simulink model "PI_VC_vs_UPI_CC_3ph_4w_v2023b"  (R2023b)
settings: Solver=FixedStepDiscrete  StartTime=0.0  StopTime=14  FixedStep=Ts_Power  MaxStep=1e-4  RelTol=1e-3
InitFcn:
  | run PI_VC_vs_UPI_CC_ini;
values from neighbouring files (symbols this model uses):
  C = 4e-6    (= 4e-06)    [PI_OL_vs_PI_CC_ini.m]    (also in PI_VC_vs_UPI_CC_ini.m)
  C_2 = 4e-6    (= 4e-06)    [PI_OL_vs_PI_CC_ini.m]    (also in PI_VC_vs_UPI_CC_ini.m)
  K_i_pll = 1.8/0.00251    (= 717.131474104)    [PI_OL_vs_PI_CC_ini.m]    (also in PI_VC_vs_UPI_CC_ini.m)
  K_p_pll = 1.8    [PI_OL_vs_PI_CC_ini.m]    (also in PI_VC_vs_UPI_CC_ini.m)
  Kp_i = 1*(L_t2 + L_s2)/tau_i    (= 2.5)    [PI_OL_vs_PI_CC_ini.m]    (also in PI_VC_vs_UPI_CC_ini.m)
  Kr_i = 2*(R_t2 + R_s2)/tau_i    (= 157.079632679)    [PI_OL_vs_PI_CC_ini.m]    (also in PI_VC_vs_UPI_CC_ini.m)
  L_line_12_13 = X_line_12_13/(2*pi*50)    (= 0.000798957814321)    [PI_OL_vs_PI_CC_ini.m]    (also in PI_VC_vs_UPI_CC_ini.m)
  L_line_13_14 = X_line_13_14/(2*pi*50)    (= 0.000200535228296)    [PI_OL_vs_PI_CC_ini.m]    (also in PI_VC_vs_UPI_CC_ini.m)
  L_n = L_t2 + L_s2    (= 0.0025)    [PI_OL_vs_PI_CC_ini.m]    (also in PI_VC_vs_UPI_CC_ini.m)
  L_s = 1.25e-3    (= 0.00125)    [PI_OL_vs_PI_CC_ini.m]    (also in PI_VC_vs_UPI_CC_ini.m)
  L_s2 = 1.25e-3    (= 0.00125)    [PI_OL_vs_PI_CC_ini.m]    (also in PI_VC_vs_UPI_CC_ini.m)
  L_t = 1.25e-3    (= 0.00125)    [PI_OL_vs_PI_CC_ini.m]    (also in PI_VC_vs_UPI_CC_ini.m)
  L_t2 = 1.25e-3    (= 0.00125)    [PI_OL_vs_PI_CC_ini.m]    (also in PI_VC_vs_UPI_CC_ini.m)
  omega = 2*pi*f    (= 314.159265359)    [PI_OL_vs_PI_CC_ini.m]    (also in PI_VC_vs_UPI_CC_ini.m)
  params_pi_cc = [S_b,U_b,K_p,T_p,K_q,T_q,X,R]    [PI_OL_vs_PI_CC_ini.m]    (also in PI_VC_vs_UPI_CC_ini.m)
  params_pi_vc = [S_b,U_b,K_p,T_p,K_q,T_q,Xv,Rv]    [PI_OL_vs_PI_CC_ini.m]    (also in PI_VC_vs_UPI_CC_ini.m)
  params_vc_cc = [R_t;L_t;R_s;L_s;K_pi;K_ii;C;K_pv;K_iv]    [PI_OL_vs_PI_CC_ini.m]    (also in PI_VC_vs_UPI_CC_ini.m)
  R_d = 10    [PI_OL_vs_PI_CC_ini.m]    (also in PI_VC_vs_UPI_CC_ini.m)
  R_d2 = 10    [PI_OL_vs_PI_CC_ini.m]    (also in PI_VC_vs_UPI_CC_ini.m)
  R_line_12_13 = (0.06)*Length    (= 0.24)    [PI_OL_vs_PI_CC_ini.m]    (also in PI_VC_vs_UPI_CC_ini.m)
  R_line_13_14 = (0.025)*Length    (= 0.1)    [PI_OL_vs_PI_CC_ini.m]    (also in PI_VC_vs_UPI_CC_ini.m)
  R_n = L_n*omega/10    (= 0.0785398163397)    [PI_OL_vs_PI_CC_ini.m]    (also in PI_VC_vs_UPI_CC_ini.m)
  R_s = L_s*omega/10    (= 0.0392699081699)    [PI_OL_vs_PI_CC_ini.m]    (also in PI_VC_vs_UPI_CC_ini.m)
  R_s2 = L_s*omega/10    (= 0.0392699081699)    [PI_OL_vs_PI_CC_ini.m]    (also in PI_VC_vs_UPI_CC_ini.m)
  R_t = L_t*omega/10    (= 0.0392699081699)    [PI_OL_vs_PI_CC_ini.m]    (also in PI_VC_vs_UPI_CC_ini.m)
  R_t2 = L_t*omega/10    (= 0.0392699081699)    [PI_OL_vs_PI_CC_ini.m]    (also in PI_VC_vs_UPI_CC_ini.m)
  S_b = 20e3    (= 20000)    [PI_OL_vs_PI_CC_ini.m]    (also in PI_VC_vs_UPI_CC_ini.m)
  Ts_Control = 50e-6    (= 5e-05)    [PI_OL_vs_PI_CC_ini.m]    (also in PI_VC_vs_UPI_CC_ini.m)
  Ts_Power = 50e-6    (= 5e-05)    [PI_OL_vs_PI_CC_ini.m]    (also in PI_VC_vs_UPI_CC_ini.m)
  v_dc = 800    [PI_OL_vs_PI_CC_ini.m]    (also in PI_VC_vs_UPI_CC_ini.m)
undefined symbols (not defined in the file or in its folder): DiscIntNeverNeededParam, omega_ref
libraries: spsFirstOrderFilterLib x32, spsUniversalBridgeLib x10, spsThreePhaseSeriesRLCBranchLib x9, spsPowerLib x6, spsThreePhaseVIMeasurementLib x6, eeGeneralControl x5, spsSeriesRLCLoadLib x5, spsRMSLib x4, spsSeriesRLCBranchLib x4, spsPower3phInstantaneousLib x3, spsThreePhaseBreakerLib x3, spsDCVoltageSourceLib x2
(part 3 of 3)

== system PI_VC_vs_UPI_CC_3ph_4w_v2023b/Control UVSG/Control corriente en alpha-beta/Resonant Controller. Impulse invariant/Subsystem1 ==
  error : Inport
  omega_PLL : Inport  Port=2
  Gain1 : Gain  Gain=Kr_i
  MATLAB Function : MATLAB Function  TreatAsAtomicUnit=on
  Unit Delay : UnitDelay  SampleTime=Ts_Control  HasFrameUpgradeWarning=on
  Unit Delay1 : UnitDelay  SampleTime=Ts_Control  HasFrameUpgradeWarning=on
  Unit Delay2 : UnitDelay  SampleTime=Ts_Control  HasFrameUpgradeWarning=on
  y : Outport
  wires:
  Gain1/1 -> MATLAB Function/2(u), Unit Delay2/1
  Unit Delay1/1 -> MATLAB Function/5(y_2)
  Unit Delay/1 -> Unit Delay1/1, MATLAB Function/4(y_1)
  omega_PLL/1 -> MATLAB Function/1(omega_vsg)
  error/1 -> Gain1/1
  MATLAB Function/1(y) -> Unit Delay/1, y/1
  Unit Delay2/1 -> MATLAB Function/3(u_1)

== system PI_VC_vs_UPI_CC_3ph_4w_v2023b/Control UVSG/Reference Computation/Transformadas Park fase/PLL ==
  v_sdq : Inport
  Demux : Demux  Outputs=2
  Discrete-Time Integrator1 : DiscreteIntegrator  SampleTime=Ts_Control  ICPrevOutput=DiscIntNeverNeededParam  ICPrevScaledInput=DiscIntNeverNeededParam
  Integrator with Wrapped State (Discrete or Continuous) : eeGeneralControl/Integrator with Wrapped State (Discrete or Continuous)  LabelModeActiveChoice=Discrete  WrappedStateUpperValue=2*pi  WrappedStateLowerValue=0  x0=0  Ts=Ts_Control
  Ki : Gain  Gain=K_i_pll
  Kp : Gain  Gain=K_p_pll
  Sum : Sum  Inputs=|++
  omega : Outport  VectorParamsAs1DForOutWhenUnconnected=off
  theta : Outport  Port=2  VectorParamsAs1DForOutWhenUnconnected=off
  wires:
  v_sdq/1 -> Demux/1
  Ki/1 -> Discrete-Time Integrator1/1
  Kp/1 -> Sum/1
  Discrete-Time Integrator1/1 -> Sum/2
  Sum/1 -> Integrator with Wrapped State (Discrete or Continuous)/1, omega/1
  Integrator with Wrapped State (Discrete or Continuous)/1 -> [theta], theta/1
  Demux/1 -> Ki/1, Kp/1

== system PI_VC_vs_UPI_CC_3ph_4w_v2023b/Control UVSG/Reference Computation/Transformadas Park fase/alpha-beta_fasea_LPF ==
  u1 : Inport
  omega : Inport  Port=2
  Gain2 : Gain  Gain=2
  MATLAB Function2 : MATLAB Function  TreatAsAtomicUnit=on
  Mux1 : Mux  Inputs=2
  Unit Delay3 : UnitDelay  SampleTime=50e-6  HasFrameUpgradeWarning=on
  Unit Delay4 : UnitDelay  SampleTime=50e-6  HasFrameUpgradeWarning=on
  Unit Delay5 : UnitDelay  SampleTime=50e-6  HasFrameUpgradeWarning=on
  "u1  " : InportShadow
  alpha_beta : Outport
  wires:
  Unit Delay3/1 -> MATLAB Function2/4(y1_k_1)
  MATLAB Function2/1(y1_k) -> Unit Delay3/1
  Unit Delay5/1 -> MATLAB Function2/2(u1_k_1)
  Unit Delay4/1 -> MATLAB Function2/5(y2_k_1)
  MATLAB Function2/2(y2_k) -> Gain2/1, Unit Delay4/1
  "u1  "/1 -> Unit Delay5/1
  omega/1 -> MATLAB Function2/3(omega)
  Gain2/1 -> Mux1/2
  u1/1 -> Mux1/1, MATLAB Function2/1(u1)
  Mux1/1 -> alpha_beta/1

== system PI_VC_vs_UPI_CC_3ph_4w_v2023b/Control UVSG/Reference Computation/Transformadas Park fase/alpha-beta_fasea_LPF1 ==
  u1 : Inport
  omega : Inport  Port=2
  Gain2 : Gain  Gain=2
  MATLAB Function2 : MATLAB Function  TreatAsAtomicUnit=on
  Mux1 : Mux  Inputs=2
  Unit Delay3 : UnitDelay  SampleTime=50e-6  HasFrameUpgradeWarning=on
  Unit Delay4 : UnitDelay  SampleTime=50e-6  HasFrameUpgradeWarning=on
  Unit Delay5 : UnitDelay  SampleTime=50e-6  HasFrameUpgradeWarning=on
  "u1  " : InportShadow
  alpha_beta : Outport
  wires:
  Mux1/1 -> alpha_beta/1
  u1/1 -> MATLAB Function2/1(u1), Mux1/1
  Gain2/1 -> Mux1/2
  omega/1 -> MATLAB Function2/3(omega)
  "u1  "/1 -> Unit Delay5/1
  MATLAB Function2/2(y2_k) -> Unit Delay4/1, Gain2/1
  Unit Delay4/1 -> MATLAB Function2/5(y2_k_1)
  Unit Delay5/1 -> MATLAB Function2/2(u1_k_1)
  MATLAB Function2/1(y1_k) -> Unit Delay3/1
  Unit Delay3/1 -> MATLAB Function2/4(y1_k_1)

== system PI_VC_vs_UPI_CC_3ph_4w_v2023b/Control UVSG/Reference Computation/Transformadas Park fase/alpha-beta_fasea_LPF2 ==
  u1 : Inport
  omega : Inport  Port=2
  Gain2 : Gain  Gain=2
  MATLAB Function2 : MATLAB Function  TreatAsAtomicUnit=on
  Mux1 : Mux  Inputs=2
  Unit Delay3 : UnitDelay  SampleTime=50e-6  HasFrameUpgradeWarning=on
  Unit Delay4 : UnitDelay  SampleTime=50e-6  HasFrameUpgradeWarning=on
  Unit Delay5 : UnitDelay  SampleTime=50e-6  HasFrameUpgradeWarning=on
  "u1  " : InportShadow
  alpha_beta : Outport
  wires:
  Unit Delay3/1 -> MATLAB Function2/4(y1_k_1)
  MATLAB Function2/1(y1_k) -> Unit Delay3/1
  Unit Delay5/1 -> MATLAB Function2/2(u1_k_1)
  Unit Delay4/1 -> MATLAB Function2/5(y2_k_1)
  MATLAB Function2/2(y2_k) -> Gain2/1, Unit Delay4/1
  "u1  "/1 -> Unit Delay5/1
  omega/1 -> MATLAB Function2/3(omega)
  Gain2/1 -> Mux1/2
  u1/1 -> Mux1/1, MATLAB Function2/1(u1)
  Mux1/1 -> alpha_beta/1

== system PI_VC_vs_UPI_CC_3ph_4w_v2023b/Control UVSG/Reference Computation/Transformadas Park fase/alpha-beta_fasea_LPF3 ==
  u1 : Inport
  omega : Inport  Port=2
  Gain2 : Gain  Gain=2
  MATLAB Function2 : MATLAB Function  TreatAsAtomicUnit=on
  Mux1 : Mux  Inputs=2
  Unit Delay3 : UnitDelay  SampleTime=50e-6  HasFrameUpgradeWarning=on
  Unit Delay4 : UnitDelay  SampleTime=50e-6  HasFrameUpgradeWarning=on
  Unit Delay5 : UnitDelay  SampleTime=50e-6  HasFrameUpgradeWarning=on
  "u1  " : InportShadow
  alpha_beta : Outport
  wires:
  Mux1/1 -> alpha_beta/1
  u1/1 -> MATLAB Function2/1(u1), Mux1/1
  Gain2/1 -> Mux1/2
  omega/1 -> MATLAB Function2/3(omega)
  "u1  "/1 -> Unit Delay5/1
  MATLAB Function2/2(y2_k) -> Unit Delay4/1, Gain2/1
  Unit Delay4/1 -> MATLAB Function2/5(y2_k_1)
  Unit Delay5/1 -> MATLAB Function2/2(u1_k_1)
  MATLAB Function2/1(y1_k) -> Unit Delay3/1
  Unit Delay3/1 -> MATLAB Function2/4(y1_k_1)

== system PI_VC_vs_UPI_CC_3ph_4w_v2023b/Control UVSG/Reference Computation/Transformadas Park fase/alpha-beta_fasea_LPF4 ==
  u1 : Inport
  omega : Inport  Port=2
  Gain2 : Gain  Gain=2
  MATLAB Function2 : MATLAB Function  TreatAsAtomicUnit=on
  Mux1 : Mux  Inputs=2
  Unit Delay3 : UnitDelay  SampleTime=50e-6  HasFrameUpgradeWarning=on
  Unit Delay4 : UnitDelay  SampleTime=50e-6  HasFrameUpgradeWarning=on
  Unit Delay5 : UnitDelay  SampleTime=50e-6  HasFrameUpgradeWarning=on
  "u1  " : InportShadow
  alpha_beta : Outport
  wires:
  Unit Delay3/1 -> MATLAB Function2/4(y1_k_1)
  MATLAB Function2/1(y1_k) -> Unit Delay3/1
  Unit Delay5/1 -> MATLAB Function2/2(u1_k_1)
  Unit Delay4/1 -> MATLAB Function2/5(y2_k_1)
  MATLAB Function2/2(y2_k) -> Gain2/1, Unit Delay4/1
  "u1  "/1 -> Unit Delay5/1
  omega/1 -> MATLAB Function2/3(omega)
  Gain2/1 -> Mux1/2
  u1/1 -> Mux1/1, MATLAB Function2/1(u1)
  Mux1/1 -> alpha_beta/1

== system PI_VC_vs_UPI_CC_3ph_4w_v2023b/Control UVSG/Reference Computation/Transformadas Park fase/alpha-beta_fasea_LPF5 ==
  u1 : Inport
  omega : Inport  Port=2
  Gain2 : Gain  Gain=2
  MATLAB Function2 : MATLAB Function  TreatAsAtomicUnit=on
  Mux1 : Mux  Inputs=2
  Unit Delay3 : UnitDelay  SampleTime=50e-6  HasFrameUpgradeWarning=on
  Unit Delay4 : UnitDelay  SampleTime=50e-6  HasFrameUpgradeWarning=on
  Unit Delay5 : UnitDelay  SampleTime=50e-6  HasFrameUpgradeWarning=on
  "u1  " : InportShadow
  alpha_beta : Outport
  wires:
  Mux1/1 -> alpha_beta/1
  u1/1 -> MATLAB Function2/1(u1), Mux1/1
  Gain2/1 -> Mux1/2
  omega/1 -> MATLAB Function2/3(omega)
  "u1  "/1 -> Unit Delay5/1
  MATLAB Function2/2(y2_k) -> Unit Delay4/1, Gain2/1
  Unit Delay4/1 -> MATLAB Function2/5(y2_k_1)
  Unit Delay5/1 -> MATLAB Function2/2(u1_k_1)
  MATLAB Function2/1(y1_k) -> Unit Delay3/1
  Unit Delay3/1 -> MATLAB Function2/4(y1_k_1)

== system PI_VC_vs_UPI_CC_3ph_4w_v2023b/Control UVSG/Reference Computation/VSG_a1/PLL ==
  v_sabc : Inport
  Demux : Demux  Outputs=2
  Discrete-Time Integrator1 : DiscreteIntegrator  InitialCondition=2*pi*50  SampleTime=Ts_Control  ICPrevOutput=DiscIntNeverNeededParam  ICPrevScaledInput=DiscIntNeverNeededParam
  Integrator with Wrapped State (Discrete or Continuous) : eeGeneralControl/Integrator with Wrapped State (Discrete or Continuous)  LabelModeActiveChoice=Discrete  WrappedStateUpperValue=2*pi  WrappedStateLowerValue=0  x0=0  Ts=Ts_Control
  Ki : Gain  Gain=K_i_pll
  Kp : Gain  Gain=K_p_pll
  MATLAB Function1 : MATLAB Function  TreatAsAtomicUnit=on
  Sum : Sum  Inputs=|++
  omega : Outport  VectorParamsAs1DForOutWhenUnconnected=off
  theta : Outport  Port=2  VectorParamsAs1DForOutWhenUnconnected=off
  wires:
  MATLAB Function1/1(dq) -> Demux/1
  v_sabc/1 -> MATLAB Function1/2(abc)
  [theta] -> MATLAB Function1/1(theta)
  Ki/1 -> Discrete-Time Integrator1/1
  Kp/1 -> Sum/1
  Discrete-Time Integrator1/1 -> Sum/2
  Sum/1 -> Integrator with Wrapped State (Discrete or Continuous)/1, omega/1
  Integrator with Wrapped State (Discrete or Continuous)/1 -> [theta], theta/1
  Demux/1 -> Ki/1, Kp/1

== system PI_VC_vs_UPI_CC_3ph_4w_v2023b/Control UVSG/Reference Computation/VSG_a2/PLL ==
  v_sabc : Inport
  Demux : Demux  Outputs=2
  Discrete-Time Integrator1 : DiscreteIntegrator  InitialCondition=2*pi*50  SampleTime=Ts_Control  ICPrevOutput=DiscIntNeverNeededParam  ICPrevScaledInput=DiscIntNeverNeededParam
  Integrator with Wrapped State (Discrete or Continuous) : eeGeneralControl/Integrator with Wrapped State (Discrete or Continuous)  LabelModeActiveChoice=Discrete  WrappedStateUpperValue=2*pi  WrappedStateLowerValue=0  x0=0  Ts=Ts_Control
  Ki : Gain  Gain=K_i_pll
  Kp : Gain  Gain=K_p_pll
  MATLAB Function1 : MATLAB Function  TreatAsAtomicUnit=on
  Sum : Sum  Inputs=|++
  omega : Outport  VectorParamsAs1DForOutWhenUnconnected=off
  theta : Outport  Port=2  VectorParamsAs1DForOutWhenUnconnected=off
  wires:
  MATLAB Function1/1(dq) -> Demux/1
  v_sabc/1 -> MATLAB Function1/2(abc)
  [theta] -> MATLAB Function1/1(theta)
  Ki/1 -> Discrete-Time Integrator1/1
  Kp/1 -> Sum/1
  Discrete-Time Integrator1/1 -> Sum/2
  Sum/1 -> Integrator with Wrapped State (Discrete or Continuous)/1, omega/1
  Integrator with Wrapped State (Discrete or Continuous)/1 -> [theta], theta/1
  Demux/1 -> Ki/1, Kp/1

== matlab function PI_VC_vs_UPI_CC_3ph_4w_v2023b/Control PI_VC/Voltage Control ==
  data: v_cdq_ref input; i_sdq input; i_tdq_ref output size=2; v_cdq input; omega input; params input; x input; dx output
function [i_tdq_ref,dx] = ctrl_vsc(v_cdq_ref,i_sdq,v_cdq,omega,params,x)

% parameters
C = params(7);
K_pv = params(8);
K_iv = params(9);

%References
v_cd_ref = v_cdq_ref(1);
v_cq_ref = v_cdq_ref(2);

i_sd = i_sdq(1);
i_sq = i_sdq(2);
v_cd = v_cdq(1);
v_cq = v_cdq(2);

% from the integrator to the states
xi_vcd = x(1);
xi_vcq = x(2);


% auxiliar
e_vcd = v_cd_ref - v_cd;
e_vcq = v_cq_ref - v_cq;

% derivatives
dxi_vcd = e_vcd;
dxi_vcq = e_vcq;


% auxiliar
u_d = K_pv*e_vcd + K_iv*xi_vcd;
u_q = K_pv*e_vcq + K_iv*xi_vcq;

% outputs
i_td_ref = (u_d - C*omega*v_cq + i_sd);
i_tq_ref = (u_q + C*omega*v_cd + i_sq);
i_tdq_ref = [i_td_ref ; i_tq_ref];


% from derivatives to the integrator
dx = [dxi_vcd;dxi_vcq];

== matlab function PI_VC_vs_UPI_CC_3ph_4w_v2023b/Control UVSG/Control corriente en alpha-beta/Resonant Controller. Impulse Invariant ==
  data: v_dc input size=1; v_salbe input size=2; eta_albe output size=2; eta_n output; u output size=2; i_sal_ref input size=1; y output size=2; u_n output; i_sbe_ref input size=1; i_salbe input size=2; omega input size=1; i_n input; i_n_ref input; u_aux_1 input size=2; y_aux_1 input size=2; y_aux_2 input size=2; u_aux_1_n input; y_aux_1_n input; y_aux_2_n input; Ts_Control parameter; Kp_i parameter; Kr_i parameter; y_aux_n output
function [eta_albe,eta_n,u,y,u_n,y_aux_n] = fcn(v_dc,v_salbe,i_sal_ref,i_sbe_ref,i_salbe,omega,i_n,i_n_ref,u_aux_1,y_aux_1,y_aux_2, u_aux_1_n, y_aux_1_n,y_aux_2_n,Ts_Control,Kp_i, Kr_i)

%Parameters

%Measurements
i_sal = i_salbe(1);
i_sbe = i_salbe(2);
v_sal = v_salbe(1);
v_sbe = v_salbe(2);

%error
e_sal = i_sal_ref - i_sal;
e_sbe = i_sbe_ref - i_sbe;

e_n = i_n_ref - i_n;


%Auxiliar
u_al = Kr_i*e_sal;
u_be = Kr_i*e_sbe;
u = [u_al;u_be];

u_n = Kr_i*e_n;

u_aux_1_al = u_aux_1(1);
u_aux_1_be = u_aux_1(2);

y_aux_1_al = y_aux_1(1);
y_aux_1_be = y_aux_1(2);

y_aux_2_al = y_aux_2(1);
y_aux_2_be = y_aux_2(2);


%Resonant controller impulse invariant
Ts = Ts_Control;
y_aux_al = u_al*Ts - u_aux_1_al*Ts*cos(omega*Ts) + 2*y_aux_1_al*cos(omega*Ts) - y_aux_2_al;
y_aux_be = u_be*Ts - u_aux_1_be*Ts*cos(omega*Ts) + 2*y_aux_1_be*cos(omega*Ts) - y_aux_2_be;

y_aux_n = u_n*Ts - u_aux_1_n*Ts*cos(omega*Ts) + 2*y_aux_1_n*cos(omega*Ts) - y_aux_2_n;

y = [y_aux_al;y_aux_be];


y_al = Kp_i*e_sal + y_aux_al;
y_be = Kp_i*e_sbe + y_aux_be;

y_n = Kp_i*e_n + y_aux_n;

%Outputs
eta_al = (y_al + v_sal)*2/v_dc;
eta_be = (y_be + v_sbe)*2/v_dc;

eta_n = (y_n)*2/v_dc;

eta_albe = [eta_al;eta_be];

== matlab function PI_VC_vs_UPI_CC_3ph_4w_v2023b/Control UVSG/Control corriente en alpha-beta/Resonant Controller. Impulse invariant/Subsystem/MATLAB Function ==
  data: omega_vsg input; y output; Ts_Control parameter; u input; u_1 input; y_1 input; y_2 input
function y  = fcn(omega_vsg, Ts_Control,u,u_1,y_1,y_2)

Ts = Ts_Control;
y = u*Ts - u_1*Ts*cos(omega_vsg*Ts) + 2*y_1*cos(omega_vsg*Ts) - y_2;

== matlab function PI_VC_vs_UPI_CC_3ph_4w_v2023b/Control UVSG/Control corriente en alpha-beta/Resonant Controller. Impulse invariant/Subsystem1/MATLAB Function ==
  data: omega_vsg input; y output; Ts_Control parameter; u input; u_1 input; y_1 input; y_2 input
function y  = fcn(omega_vsg, Ts_Control,u,u_1,y_1,y_2)

Ts = Ts_Control;
y = u*Ts - u_1*Ts*cos(omega_vsg*Ts) + 2*y_1*cos(omega_vsg*Ts) - y_2;

== matlab function PI_VC_vs_UPI_CC_3ph_4w_v2023b/Control UVSG/PARK_PLL/MATLAB Function1 ==
  data: theta input size=1; dq output; abc input
function dq  = fcn(theta,abc)
%#codegen

T_p = 2.0/3.0*[[ cos(theta), cos(theta-2.0/3.0*pi), cos(theta+2.0/3.0*pi)];
               [-sin(theta),-sin(theta-2.0/3.0*pi),-sin(theta+2.0/3.0*pi)]];
           
dq=T_p*abc;

== matlab function PI_VC_vs_UPI_CC_3ph_4w_v2023b/Control UVSG/PARK_PLL/MATLAB Function2 ==
  data: theta input size=1; dq output; abc input
function dq  = fcn(theta,abc)
%#codegen

T_p = 2.0/3.0*[[ cos(theta), cos(theta-2.0/3.0*pi), cos(theta+2.0/3.0*pi)];
               [-sin(theta),-sin(theta-2.0/3.0*pi),-sin(theta+2.0/3.0*pi)]];
           
dq=T_p*abc;

== matlab function PI_VC_vs_UPI_CC_3ph_4w_v2023b/Control UVSG/Control corriente en alpha-beta/Resonant Controller. Impulse Invariant1 ==
  data: v_dc input size=1; v_salbe input size=2; eta_albe output size=2; eta_n output; u output size=2; i_sal_ref input size=1; y output size=2; u_n output; i_sbe_ref input size=1; i_salbe input size=2; omega input size=1; i_n input; i_n_ref input; u_aux_1 input size=2; y_aux_1 input size=2; y_aux_2 input size=2; u_aux_1_n input; y_aux_1_n input; y_aux_2_n input; Ts_Control parameter; Kp_i parameter; Kr_i parameter; y_aux_n output
function [eta_albe,eta_n,u,y,u_n,y_aux_n] = fcn(v_dc,v_salbe,i_sal_ref,i_sbe_ref,i_salbe,omega,i_n,i_n_ref,u_aux_1,y_aux_1,y_aux_2, u_aux_1_n, y_aux_1_n,y_aux_2_n,Ts_Control,Kp_i, Kr_i)

%Parameters

%Measurements
i_sal = i_salbe(1);
i_sbe = i_salbe(2);
v_sal = v_salbe(1);
v_sbe = v_salbe(2);

%error
e_sal = i_sal_ref - i_sal;
e_sbe = i_sbe_ref - i_sbe;

e_n = i_n_ref - i_n;


%Auxiliar
u_al = Kr_i*e_sal;
u_be = Kr_i*e_sbe;
u = [u_al;u_be];

u_n = Kr_i*e_n;

u_aux_1_al = u_aux_1(1);
u_aux_1_be = u_aux_1(2);

y_aux_1_al = y_aux_1(1);
y_aux_1_be = y_aux_1(2);

y_aux_2_al = y_aux_2(1);
y_aux_2_be = y_aux_2(2);


%Resonant controller impulse invariant
Ts = Ts_Control;
y_aux_al = u_al*Ts - u_aux_1_al*Ts*cos(omega*Ts) + 2*y_aux_1_al*cos(omega*Ts) - y_aux_2_al;
y_aux_be = u_be*Ts - u_aux_1_be*Ts*cos(omega*Ts) + 2*y_aux_1_be*cos(omega*Ts) - y_aux_2_be;

y_aux_n = u_n*Ts - u_aux_1_n*Ts*cos(omega*Ts) + 2*y_aux_1_n*cos(omega*Ts) - y_aux_2_n;

y = [y_aux_al;y_aux_be];


y_al = Kp_i*e_sal + y_aux_al;
y_be = Kp_i*e_sbe + y_aux_be;

y_n = Kp_i*e_n + y_aux_n;

%Outputs
eta_al = (y_al + v_sal)*2/v_dc;
eta_be = (y_be + v_sbe)*2/v_dc;

eta_n = (y_n)*2/v_dc;

eta_albe = [eta_al;eta_be];

== matlab function PI_VC_vs_UPI_CC_3ph_4w_v2023b/Control UVSG/PARK_PLL/MATLAB Function3 ==
  data: theta input size=1; dq output; abc input
function dq  = fcn(theta,abc)
%#codegen

T_p = 2.0/3.0*[[ cos(theta), cos(theta-2.0/3.0*pi), cos(theta+2.0/3.0*pi)];
               [-sin(theta),-sin(theta-2.0/3.0*pi),-sin(theta+2.0/3.0*pi)]];
           
dq=T_p*abc;

== matlab function PI_VC_vs_UPI_CC_3ph_4w_v2023b/Control UVSG/PARK_PLL/MATLAB Function5 ==
  data: theta input size=1; abc output size=3; dq input
function abc  = fcn(theta,dq)
%#codegen

T_p_inv = [[            cos(theta),            -sin(theta)];
           [ cos(theta-2.0/3.0*pi), -sin(theta-2.0/3.0*pi)];
           [ cos(theta+2.0/3.0*pi), -sin(theta+2.0/3.0*pi)]];
           
abc=T_p_inv*dq;

== matlab function PI_VC_vs_UPI_CC_3ph_4w_v2023b/Control UVSG/PARK_PLL/PLL/MATLAB Function1 ==
  data: theta input size=1; dq output; abc input
function dq  = fcn(theta,abc)
%#codegen

T_p = 2.0/3.0*[[ cos(theta), cos(theta-2.0/3.0*pi), cos(theta+2.0/3.0*pi)];
               [-sin(theta),-sin(theta-2.0/3.0*pi),-sin(theta+2.0/3.0*pi)]];
           
dq=T_p*abc;

== matlab function PI_VC_vs_UPI_CC_3ph_4w_v2023b/Control UVSG/Reference Computation/MATLAB Function1 ==
  data: albe input size=2; a output size=1
function a  = fcn(albe)
%#codegen
theta = 0;
a=cos(theta)*albe(1) - sin(theta)*albe(2) ;

== matlab function PI_VC_vs_UPI_CC_3ph_4w_v2023b/Control UVSG/Reference Computation/MATLAB Function2 ==
  data: albe input size=2; a output size=1
function a  = fcn(albe)
%#codegen
theta = 0;
a=cos(theta)*albe(1) - sin(theta)*albe(2) ;

== matlab function PI_VC_vs_UPI_CC_3ph_4w_v2023b/Control UVSG/Reference Computation/MATLAB Function5 ==
  data: albe input size=2; a output size=1
function a  = fcn(albe)
%#codegen
theta = 0;
a=cos(theta)*albe(1) - sin(theta)*albe(2) ;

== matlab function PI_VC_vs_UPI_CC_3ph_4w_v2023b/Control UVSG/Reference Computation/Transformadas Park fase/MATLAB Function1 ==
  data: alpha_beta input size=2; dq output; theta input
function dq = fcn(alpha_beta,theta)
alpha = alpha_beta(1);
beta = alpha_beta(2);

d= alpha*cos(theta)+ beta*sin(theta);
q= -alpha*sin(theta) + beta*cos(theta);
dq = [d;q];

== matlab function PI_VC_vs_UPI_CC_3ph_4w_v2023b/Control UVSG/Reference Computation/Transformadas Park fase/MATLAB Function2 ==
  data: alpha_beta input size=2; dq output; theta input
function dq = fcn(alpha_beta,theta)
alpha = alpha_beta(1);
beta = alpha_beta(2);

d= alpha*cos(theta)+ beta*sin(theta);
q= -alpha*sin(theta) + beta*cos(theta);
dq = [d;q];

== matlab function PI_VC_vs_UPI_CC_3ph_4w_v2023b/Control UVSG/Reference Computation/Transformadas Park fase/MATLAB Function3 ==
  data: alpha_beta input size=2; dq output; theta input
function dq = fcn(alpha_beta,theta)
alpha = alpha_beta(1);
beta = alpha_beta(2);

d= alpha*cos(theta)+ beta*sin(theta);
q= -alpha*sin(theta) + beta*cos(theta);
dq = [d;q];

== matlab function PI_VC_vs_UPI_CC_3ph_4w_v2023b/Control PI_VC/Current Control ==
  data: i_tdq_ref input; i_tdq input; eta_dq output size=2; v_cdq input; v_dc input; omega input; params input; x input; dx output
function [eta_dq,dx] = ctrl_vsc(i_tdq_ref,i_tdq,v_cdq,v_dc,omega,params,x)

% parameters
L_t = params(2);
K_pi = params(5);
K_ii = params(6);

%References
i_td_ref = i_tdq_ref(1);
i_tq_ref = i_tdq_ref(2);

i_td = i_tdq(1);
i_tq = i_tdq(2);
v_cd = v_cdq(1);
v_cq = v_cdq(2);

% from the integrator to the states
xi_itd = x(1);
xi_itq = x(2);


% auxiliar
e_itd = i_td_ref - i_td;
e_itq = i_tq_ref - i_tq;

% derivatives
dxi_itd = e_itd;
dxi_itq = e_itq;


% auxiliar
u_d = K_pi*e_itd + K_ii*xi_itd;
u_q = K_pi*e_itq + K_ii*xi_itq;
L = L_t;

% outputs
eta_d = 2/v_dc*(u_d - L*omega*i_tq + v_cd);
eta_q = 2/v_dc*(u_q + L*omega*i_td + v_cq);
eta_dq = [eta_d ; eta_q];


% from derivatives to the integrator
dx = [dxi_itd;dxi_itq];

== matlab function PI_VC_vs_UPI_CC_3ph_4w_v2023b/Control UVSG/Reference Computation/Transformadas Park fase/alpha-beta_fasea_LPF/MATLAB Function2 ==
  data: u1 input; u1_k_1 input; omega input; y1_k_1 input; y1_k output; y2_k_1 input; y2_k output
function [y1_k,y2_k]  = fcn(u1,u1_k_1,omega,y1_k_1,y2_k_1)


Ts_Control = 50e-6;
%y = x
%y1_k = (u1*omega + exp(-omega)*y1_k_1);
y1_k = ((u1 + u1_k_1)*omega*Ts_Control - (omega*Ts_Control-2)*y1_k_1)/(omega*Ts_Control + 2);

u2 = y1_k;
u2_k_1 = y1_k_1;

%y2_k = (u2*omega + exp(-omega)*y2_k_1);
y2_k = ((u2 + u2_k_1)*omega*Ts_Control - (omega*Ts_Control-2)*y2_k_1)/(omega*Ts_Control + 2);

== matlab function PI_VC_vs_UPI_CC_3ph_4w_v2023b/Control UVSG/Reference Computation/Transformadas Park fase/alpha-beta_fasea_LPF1/MATLAB Function2 ==
  data: u1 input; u1_k_1 input; omega input; y1_k_1 input; y1_k output; y2_k_1 input; y2_k output
function [y1_k,y2_k]  = fcn(u1,u1_k_1,omega,y1_k_1,y2_k_1)


Ts_Control = 50e-6;
%y = x
%y1_k = (u1*omega + exp(-omega)*y1_k_1);
y1_k = ((u1 + u1_k_1)*omega*Ts_Control - (omega*Ts_Control-2)*y1_k_1)/(omega*Ts_Control + 2);

u2 = y1_k;
u2_k_1 = y1_k_1;

%y2_k = (u2*omega + exp(-omega)*y2_k_1);
y2_k = ((u2 + u2_k_1)*omega*Ts_Control - (omega*Ts_Control-2)*y2_k_1)/(omega*Ts_Control + 2);

== matlab function PI_VC_vs_UPI_CC_3ph_4w_v2023b/Control UVSG/Reference Computation/Transformadas Park fase/alpha-beta_fasea_LPF2/MATLAB Function2 ==
  data: u1 input; u1_k_1 input; omega input; y1_k_1 input; y1_k output; y2_k_1 input; y2_k output
function [y1_k,y2_k]  = fcn(u1,u1_k_1,omega,y1_k_1,y2_k_1)


Ts_Control = 50e-6;
%y = x
%y1_k = (u1*omega + exp(-omega)*y1_k_1);
y1_k = ((u1 + u1_k_1)*omega*Ts_Control - (omega*Ts_Control-2)*y1_k_1)/(omega*Ts_Control + 2);

u2 = y1_k;
u2_k_1 = y1_k_1;

%y2_k = (u2*omega + exp(-omega)*y2_k_1);
y2_k = ((u2 + u2_k_1)*omega*Ts_Control - (omega*Ts_Control-2)*y2_k_1)/(omega*Ts_Control + 2);

== matlab function PI_VC_vs_UPI_CC_3ph_4w_v2023b/Control UVSG/Reference Computation/Transformadas Park fase/MATLAB Function ==
  data: v_salbe_a input size=2; p output; i_salbe_a input size=2; q output
function [p,q] = fcn(v_salbe_a,i_salbe_a)

vs_al = v_salbe_a(1);
vs_be = v_salbe_a(2);
is_al = i_salbe_a(1);
is_be = i_salbe_a(2);
p=3/2*(vs_al*is_al + vs_be*is_be);
q=-3/2*(vs_al*is_be - vs_be*is_al);

== matlab function PI_VC_vs_UPI_CC_3ph_4w_v2023b/Control UVSG/Reference Computation/Transformadas Park fase/MATLAB Function4 ==
  data: v_salbe_a input size=2; p output; i_salbe_a input size=2; q output
function [p,q] = fcn(v_salbe_a,i_salbe_a)

vs_al = v_salbe_a(1);
vs_be = v_salbe_a(2);
is_al = i_salbe_a(1);
is_be = i_salbe_a(2);
p=3/2*(vs_al*is_al + vs_be*is_be);
q=-3/2*(vs_al*is_be - vs_be*is_al);

== matlab function PI_VC_vs_UPI_CC_3ph_4w_v2023b/Control UVSG/Reference Computation/Transformadas Park fase/MATLAB Function5 ==
  data: v_salbe_a input size=2; p output; i_salbe_a input size=2; q output
function [p,q] = fcn(v_salbe_a,i_salbe_a)

vs_al = v_salbe_a(1);
vs_be = v_salbe_a(2);
is_al = i_salbe_a(1);
is_be = i_salbe_a(2);
p=3/2*(vs_al*is_al + vs_be*is_be);
q=-3/2*(vs_al*is_be - vs_be*is_al);

== matlab function PI_VC_vs_UPI_CC_3ph_4w_v2023b/Control UVSG/Reference Computation/Transformadas Park fase/alpha-beta_fasea_LPF3/MATLAB Function2 ==
  data: u1 input; u1_k_1 input; omega input; y1_k_1 input; y1_k output; y2_k_1 input; y2_k output
function [y1_k,y2_k]  = fcn(u1,u1_k_1,omega,y1_k_1,y2_k_1)


Ts_Control = 50e-6;
%y = x
%y1_k = (u1*omega + exp(-omega)*y1_k_1);
y1_k = ((u1 + u1_k_1)*omega*Ts_Control - (omega*Ts_Control-2)*y1_k_1)/(omega*Ts_Control + 2);

u2 = y1_k;
u2_k_1 = y1_k_1;

%y2_k = (u2*omega + exp(-omega)*y2_k_1);
y2_k = ((u2 + u2_k_1)*omega*Ts_Control - (omega*Ts_Control-2)*y2_k_1)/(omega*Ts_Control + 2);

== matlab function PI_VC_vs_UPI_CC_3ph_4w_v2023b/Control UVSG/Reference Computation/Transformadas Park fase/alpha-beta_fasea_LPF4/MATLAB Function2 ==
  data: u1 input; u1_k_1 input; omega input; y1_k_1 input; y1_k output; y2_k_1 input; y2_k output
function [y1_k,y2_k]  = fcn(u1,u1_k_1,omega,y1_k_1,y2_k_1)


Ts_Control = 50e-6;
%y = x
%y1_k = (u1*omega + exp(-omega)*y1_k_1);
y1_k = ((u1 + u1_k_1)*omega*Ts_Control - (omega*Ts_Control-2)*y1_k_1)/(omega*Ts_Control + 2);

u2 = y1_k;
u2_k_1 = y1_k_1;

%y2_k = (u2*omega + exp(-omega)*y2_k_1);
y2_k = ((u2 + u2_k_1)*omega*Ts_Control - (omega*Ts_Control-2)*y2_k_1)/(omega*Ts_Control + 2);

== matlab function PI_VC_vs_UPI_CC_3ph_4w_v2023b/Control UVSG/Reference Computation/Transformadas Park fase/alpha-beta_fasea_LPF5/MATLAB Function2 ==
  data: u1 input; u1_k_1 input; omega input; y1_k_1 input; y1_k output; y2_k_1 input; y2_k output
function [y1_k,y2_k]  = fcn(u1,u1_k_1,omega,y1_k_1,y2_k_1)


Ts_Control = 50e-6;
%y = x
%y1_k = (u1*omega + exp(-omega)*y1_k_1);
y1_k = ((u1 + u1_k_1)*omega*Ts_Control - (omega*Ts_Control-2)*y1_k_1)/(omega*Ts_Control + 2);

u2 = y1_k;
u2_k_1 = y1_k_1;

%y2_k = (u2*omega + exp(-omega)*y2_k_1);
y2_k = ((u2 + u2_k_1)*omega*Ts_Control - (omega*Ts_Control-2)*y2_k_1)/(omega*Ts_Control + 2);

== matlab function PI_VC_vs_UPI_CC_3ph_4w_v2023b/Control UVSG/Reference Computation/VSG_a/MATLAB Function1 ==
  data: theta input size=1; dq output; abc input
function dq  = fcn(theta,abc)
%#codegen

T_p = 2.0/3.0*[[ cos(theta), cos(theta-2.0/3.0*pi), cos(theta+2.0/3.0*pi)];
               [-sin(theta),-sin(theta-2.0/3.0*pi),-sin(theta+2.0/3.0*pi)]];
           
dq=T_p*abc;

== matlab function PI_VC_vs_UPI_CC_3ph_4w_v2023b/Control UVSG/Reference Computation/VSG_a/MATLAB Function2 ==
  data: alpha_beta input size=2; dq output; theta input
function dq = fcn(alpha_beta,theta)
alpha = alpha_beta(1);
beta = alpha_beta(2);

d= alpha*cos(theta)+ beta*sin(theta);
q= -alpha*sin(theta) + beta*cos(theta);
dq = [d;q];

== matlab function PI_VC_vs_UPI_CC_3ph_4w_v2023b/Control UVSG/Reference Computation/VSG_a/MATLAB Function3 ==
  data: theta input size=1; abc output size=3; dq input
function abc  = fcn(theta,dq)
%#codegen

T_p_inv = [[            cos(theta),            -sin(theta)];
           [ cos(theta-2.0/3.0*pi), -sin(theta-2.0/3.0*pi)];
           [ cos(theta+2.0/3.0*pi), -sin(theta+2.0/3.0*pi)]];
           
abc=T_p_inv*dq;

== matlab function PI_VC_vs_UPI_CC_3ph_4w_v2023b/Control UVSG/Reference Computation/VSG_a/MATLAB Function4 ==
  data: alpha_beta input size=2; dq output; theta input
function dq = fcn(alpha_beta,theta)
alpha = alpha_beta(1);
beta = alpha_beta(2);

d= alpha*cos(theta)+ beta*sin(theta);
q= -alpha*sin(theta) + beta*cos(theta);
dq = [d;q];

== matlab function PI_VC_vs_UPI_CC_3ph_4w_v2023b/Control UVSG/Reference Computation/VSG_a/VSG ==
  data: p_m_ref input; q_s_ref input; p input; q input; i_sdq input; i_sdq_ref output size=2; omega_rads output; v_sdq input; params input; omega_base input; x input; dx output
function [i_sdq_ref,omega_rads,dx] = ctrl_3(p_m_ref,q_s_ref,p,q,i_sdq,v_sdq,params,omega_base,x)
%Initialization
i_sdq_ref = [0;0];
fault_flag = 0;
e_0 = 1.0;

% parameters
S_b = params(1);
U_b = params(2);
K_p = params(3);
T_p = params(4);
K_q = params(5);
T_q = params(6);
X = params(7);
R = params(8);

%Base value
I_b = S_b/(sqrt(3)*U_b);
I_bdq = I_b*sqrt(2); 
U_bdq = U_b*(sqrt(2/3));

%Current and voltage in pu
v_sd = v_sdq(1)/U_bdq; % input in SI that is coverted to pu
v_sq = v_sdq(2)/U_bdq; % input in SI that is coverted to pu
i_sd = i_sdq(1)/I_bdq; % input in SI that is coverted to pu
i_sq = i_sdq(2)/I_bdq; % input in SI that is coverted to pu
%Active power en pu
p_s = i_sd*v_sd + i_sq*v_sq; % pu
q_s = i_sd*v_sq - i_sq*v_sd; % pu 

% from the integrator to the states
phi  = x(1);
xi_p = x(2);
xi_q = x(3);
omega_fil = x(4);

%error of active and reactive power
epsilon_p = (p_m_ref - p_s)*(1.0-fault_flag);
epsilon_q = q_s_ref - q_s;

%omega VSG
omega = K_p*(epsilon_p + xi_p/T_p) + omega_base; 
omega_rads = 2.0*pi*50.0*omega;
%Derivative outputs
dphi =  omega_rads;
dxi_p = epsilon_p;
dxi_q = epsilon_q; 
domega_rads = 1.0/1.0*(2.0*pi*50.0*omega - omega_fil);

%Voltage increase
DV =   K_q*(epsilon_q + xi_q/T_q); 

%Saturation of DV
DV_sat = DV;
if DV_sat > 0.1 
    DV_sat = 0.1;
    dxi_q = 0.0;
end
if DV_sat < -0.1 
    DV_sat = -0.1;
    dxi_q = 0.0;
end   

%Electromotive force of VSG
e = e_0 + DV_sat; 

%Virtual impdance
i_sd = -(X*e + R*v_sd + X*v_sq)/(R^2 + X^2);
i_sq = -(R*e + R*v_sq - X*v_sd)/(R^2 + X^2);

%Current references in A
i_sdq_ref(1) = i_sd*I_bdq;
i_sdq_ref(2) = i_sq*I_bdq;


% from derivatives to the integrator
dx = [dphi;dxi_p;dxi_q;domega_rads];

== matlab function PI_VC_vs_UPI_CC_3ph_4w_v2023b/Control PI_VC/PLL/MATLAB Function1 ==
  data: theta input size=1; dq output; abc input
function dq  = fcn(theta,abc)
%#codegen

T_p = 2.0/3.0*[[ cos(theta), cos(theta-2.0/3.0*pi), cos(theta+2.0/3.0*pi)];
               [-sin(theta),-sin(theta-2.0/3.0*pi),-sin(theta+2.0/3.0*pi)]];
           
dq=T_p*abc;

== matlab function PI_VC_vs_UPI_CC_3ph_4w_v2023b/Control UVSG/Reference Computation/Transformadas Park fase/MATLAB Function6 ==
  data: i_sabc input; pa output; v_sabc input; qa output; pb output; qb output; pc output; qc output
function [pa,qa,pb,qb,pc,qc] = fcn(i_sabc,v_sabc)

ia = i_sabc(1);
ib = i_sabc(2);
ic = i_sabc(3);

va = v_sabc(1);
vb = v_sabc(2);
vc = v_sabc(3);

pa = ia*va;
qa = 1/sqrt(3)*ia*(vb - vc);

pb = ib*vb;
qb = 1/sqrt(3)*ib*(vc -va);

pc = ic*vc;
qc = 1/sqrt(3)*ic*(va -vb);

== matlab function PI_VC_vs_UPI_CC_3ph_4w_v2023b/Control UVSG/Reference Computation/VSG_a1/MATLAB Function1 ==
  data: theta input size=1; dq output; abc input
function dq  = fcn(theta,abc)
%#codegen

T_p = 2.0/3.0*[[ cos(theta), cos(theta-2.0/3.0*pi), cos(theta+2.0/3.0*pi)];
               [-sin(theta),-sin(theta-2.0/3.0*pi),-sin(theta+2.0/3.0*pi)]];
           
dq=T_p*abc;

== matlab function PI_VC_vs_UPI_CC_3ph_4w_v2023b/Control UVSG/Reference Computation/VSG_a1/MATLAB Function2 ==
  data: alpha_beta input size=2; dq output; theta input
function dq = fcn(alpha_beta,theta)
alpha = alpha_beta(1);
beta = alpha_beta(2);

d= alpha*cos(theta)+ beta*sin(theta);
q= -alpha*sin(theta) + beta*cos(theta);
dq = [d;q];

== matlab function PI_VC_vs_UPI_CC_3ph_4w_v2023b/Control UVSG/Reference Computation/VSG_a1/MATLAB Function3 ==
  data: theta input size=1; abc output size=3; dq input
function abc  = fcn(theta,dq)
%#codegen

T_p_inv = [[            cos(theta),            -sin(theta)];
           [ cos(theta-2.0/3.0*pi), -sin(theta-2.0/3.0*pi)];
           [ cos(theta+2.0/3.0*pi), -sin(theta+2.0/3.0*pi)]];
           
abc=T_p_inv*dq;

== matlab function PI_VC_vs_UPI_CC_3ph_4w_v2023b/Control UVSG/Reference Computation/VSG_a1/MATLAB Function4 ==
  data: alpha_beta input size=2; dq output; theta input
function dq = fcn(alpha_beta,theta)
alpha = alpha_beta(1);
beta = alpha_beta(2);

d= alpha*cos(theta)+ beta*sin(theta);
q= -alpha*sin(theta) + beta*cos(theta);
dq = [d;q];

== matlab function PI_VC_vs_UPI_CC_3ph_4w_v2023b/Control UVSG/Reference Computation/VSG_a1/VSG ==
  data: p_m_ref input; q_s_ref input; p input; q input; i_sdq input; i_sdq_ref output size=2; omega_rads output; v_sdq input; params input; omega_base input; x input; dx output
function [i_sdq_ref,omega_rads,dx] = ctrl_3(p_m_ref,q_s_ref,p,q,i_sdq,v_sdq,params,omega_base,x)
%Initialization
i_sdq_ref = [0;0];
fault_flag = 0;
e_0 = 1.0;

% parameters
S_b = params(1);
U_b = params(2);
K_p = params(3);
T_p = params(4);
K_q = params(5);
T_q = params(6);
X = params(7);
R = params(8);

%Base value
I_b = S_b/(sqrt(3)*U_b);
I_bdq = I_b*sqrt(2); 
U_bdq = U_b*(sqrt(2/3));

%Current and voltage in pu
v_sd = v_sdq(1)/U_bdq; % input in SI that is coverted to pu
v_sq = v_sdq(2)/U_bdq; % input in SI that is coverted to pu
i_sd = i_sdq(1)/I_bdq; % input in SI that is coverted to pu
i_sq = i_sdq(2)/I_bdq; % input in SI that is coverted to pu
%Active power en pu
p_s = i_sd*v_sd + i_sq*v_sq; % pu
q_s = i_sd*v_sq - i_sq*v_sd; % pu 

% from the integrator to the states
phi  = x(1);
xi_p = x(2);
xi_q = x(3);
omega_fil = x(4);

%error of active and reactive power
epsilon_p = (p_m_ref - p_s)*(1.0-fault_flag);
epsilon_q = q_s_ref - q_s;

%omega VSG
omega = K_p*(epsilon_p + xi_p/T_p) + omega_base; 
omega_rads = 2.0*pi*50.0*omega;
%Derivative outputs
dphi =  omega_rads;
dxi_p = epsilon_p;
dxi_q = epsilon_q; 
domega_rads = 1.0/1.0*(2.0*pi*50.0*omega - omega_fil);

%Voltage increase
DV =   K_q*(epsilon_q + xi_q/T_q); 

%Saturation of DV
DV_sat = DV;
if DV_sat > 0.1 
    DV_sat = 0.1;
    dxi_q = 0.0;
end
if DV_sat < -0.1 
    DV_sat = -0.1;
    dxi_q = 0.0;
end   

%Electromotive force of VSG
e = e_0 + DV_sat; 

%Virtual impdance
i_sd = -(X*e + R*v_sd + X*v_sq)/(R^2 + X^2);
i_sq = -(R*e + R*v_sq - X*v_sd)/(R^2 + X^2);

%Current references in A
i_sdq_ref(1) = i_sd*I_bdq;
i_sdq_ref(2) = i_sq*I_bdq;


% from derivatives to the integrator
dx = [dphi;dxi_p;dxi_q;domega_rads];

== matlab function PI_VC_vs_UPI_CC_3ph_4w_v2023b/Control UVSG/Reference Computation/VSG_a2/MATLAB Function1 ==
  data: theta input size=1; dq output; abc input
function dq  = fcn(theta,abc)
%#codegen

T_p = 2.0/3.0*[[ cos(theta), cos(theta-2.0/3.0*pi), cos(theta+2.0/3.0*pi)];
               [-sin(theta),-sin(theta-2.0/3.0*pi),-sin(theta+2.0/3.0*pi)]];
           
dq=T_p*abc;

== matlab function PI_VC_vs_UPI_CC_3ph_4w_v2023b/Control PI_VC/VSG ==
  data: e_0 input; p_m_ref input; q_s_ref input; i_sdq input; v_sdq input; v_mdq_ref output size=2; omega_rads output; params input; omega_base input; x input; dx output
function [v_mdq_ref,omega_rads,dx] = ctrl_3(e_0,p_m_ref,q_s_ref,i_sdq,v_sdq,params,omega_base,x)
%Initialization
v_mdq_ref = [0;0];
fault_flag = 0;

% parameters
S_b = params(1);
U_b = params(2);
K_p = params(3);
T_p = params(4);
K_q = params(5);
T_q = params(6);
X = params(7);
R = params(8);

%Base value
I_b = S_b/(sqrt(3)*U_b);
I_bdq = I_b*sqrt(2); 
U_bdq = U_b*(sqrt(2/3));

%Current and voltage in pu

v_sd = v_sdq(1)/U_bdq; % input in SI that is coverted to pu
v_sq = v_sdq(2)/U_bdq; % input in SI that is coverted to pu
i_sd = i_sdq(1)/I_bdq; % input in SI that is coverted to pu
i_sq = i_sdq(2)/I_bdq; % input in SI that is coverted to pu
%Active power en pu
p_s = i_sd*v_sd + i_sq*v_sq; % pu
q_s = i_sd*v_sq - i_sq*v_sd; % pu 

% from the integrator to the states
phi  = x(1);
xi_p = x(2);
xi_q = x(3);
omega_fil = x(4);

%error of active and reactive power
epsilon_p = (p_m_ref - p_s)*(1.0-fault_flag);
epsilon_q = q_s_ref - q_s;

%omega VSG
omega = K_p*(epsilon_p + xi_p/T_p) + omega_base; 
omega_rads = 2.0*pi*50.0*omega;
%Derivative outputs
dphi =  omega_rads;
dxi_p = epsilon_p;
dxi_q = epsilon_q; 
domega_rads = 1.0/1.0*(2.0*pi*50.0*omega - omega_fil);

%Voltage increase
DV =   K_q*(epsilon_q + xi_q/T_q*1); 

%Saturation of DV
DV_sat = DV;
if DV_sat > 0.1 
    DV_sat = 0.1;
    dxi_q = 0.0;
end
if DV_sat < -0.1 
    DV_sat = -0.1;
    dxi_q = 0.0;
end   

%Electromotive force of VSG
e = e_0 + DV_sat; 
e_d =0;
e_q = -e;
%Virtual impdance
v_md = e_d - (R*i_sd - X*i_sq) ;
v_mq = e_q - (X*i_sd + R*i_sq) ;

%Current references in A
v_mdq_ref(1) = v_md*U_bdq;
v_mdq_ref(2) = v_mq*U_bdq;


% from derivatives to the integrator
dx = [dphi;dxi_p;dxi_q;domega_rads];

== matlab function PI_VC_vs_UPI_CC_3ph_4w_v2023b/Control UVSG/Reference Computation/VSG_a2/MATLAB Function2 ==
  data: alpha_beta input size=2; dq output; theta input
function dq = fcn(alpha_beta,theta)
alpha = alpha_beta(1);
beta = alpha_beta(2);

d= alpha*cos(theta)+ beta*sin(theta);
q= -alpha*sin(theta) + beta*cos(theta);
dq = [d;q];

== matlab function PI_VC_vs_UPI_CC_3ph_4w_v2023b/Control UVSG/Reference Computation/VSG_a1/PLL/MATLAB Function1 ==
  data: theta input size=1; dq output; abc input
function dq  = fcn(theta,abc)
%#codegen

T_p = 2.0/3.0*[[ cos(theta), cos(theta-2.0/3.0*pi), cos(theta+2.0/3.0*pi)];
               [-sin(theta),-sin(theta-2.0/3.0*pi),-sin(theta+2.0/3.0*pi)]];
           
dq=T_p*abc;

== matlab function PI_VC_vs_UPI_CC_3ph_4w_v2023b/Control UVSG/Reference Computation/VSG_a1/MATLAB Function5 ==
  data: theta input size=1; abc output size=3; dq input
function abc  = fcn(theta,dq)
%#codegen

T_p_inv = [[            cos(theta),            -sin(theta)];
           [ cos(theta-2.0/3.0*pi), -sin(theta-2.0/3.0*pi)];
           [ cos(theta+2.0/3.0*pi), -sin(theta+2.0/3.0*pi)]];
           
abc=T_p_inv*dq;

== matlab function PI_VC_vs_UPI_CC_3ph_4w_v2023b/Control UVSG/Reference Computation/VSG_a2/MATLAB Function3 ==
  data: theta input size=1; abc output size=3; dq input
function abc  = fcn(theta,dq)
%#codegen

T_p_inv = [[            cos(theta),            -sin(theta)];
           [ cos(theta-2.0/3.0*pi), -sin(theta-2.0/3.0*pi)];
           [ cos(theta+2.0/3.0*pi), -sin(theta+2.0/3.0*pi)]];
           
abc=T_p_inv*dq;

== matlab function PI_VC_vs_UPI_CC_3ph_4w_v2023b/Control UVSG/Reference Computation/VSG_a2/MATLAB Function4 ==
  data: alpha_beta input size=2; dq output; theta input
function dq = fcn(alpha_beta,theta)
alpha = alpha_beta(1);
beta = alpha_beta(2);

d= alpha*cos(theta)+ beta*sin(theta);
q= -alpha*sin(theta) + beta*cos(theta);
dq = [d;q];

== matlab function PI_VC_vs_UPI_CC_3ph_4w_v2023b/Control UVSG/Reference Computation/VSG_a2/MATLAB Function5 ==
  data: theta input size=1; abc output size=3; dq input
function abc  = fcn(theta,dq)
%#codegen

T_p_inv = [[            cos(theta),            -sin(theta)];
           [ cos(theta-2.0/3.0*pi), -sin(theta-2.0/3.0*pi)];
           [ cos(theta+2.0/3.0*pi), -sin(theta+2.0/3.0*pi)]];
           
abc=T_p_inv*dq;

== matlab function PI_VC_vs_UPI_CC_3ph_4w_v2023b/Control UVSG/Reference Computation/VSG_a2/PLL/MATLAB Function1 ==
  data: theta input size=1; dq output; abc input
function dq  = fcn(theta,abc)
%#codegen

T_p = 2.0/3.0*[[ cos(theta), cos(theta-2.0/3.0*pi), cos(theta+2.0/3.0*pi)];
               [-sin(theta),-sin(theta-2.0/3.0*pi),-sin(theta+2.0/3.0*pi)]];
           
dq=T_p*abc;

== matlab function PI_VC_vs_UPI_CC_3ph_4w_v2023b/Control UVSG/Reference Computation/VSG_a2/VSG ==
  data: p_m_ref input; q_s_ref input; p input; q input; i_sdq input; i_sdq_ref output size=2; omega_rads output; v_sdq input; params input; omega_base input; x input; dx output
function [i_sdq_ref,omega_rads,dx] = ctrl_3(p_m_ref,q_s_ref,p,q,i_sdq,v_sdq,params,omega_base,x)
%Initialization
i_sdq_ref = [0;0];
fault_flag = 0;
e_0 = 1.0;

% parameters
S_b = params(1);
U_b = params(2);
K_p = params(3);
T_p = params(4);
K_q = params(5);
T_q = params(6);
X = params(7);
R = params(8);

%Base value
I_b = S_b/(sqrt(3)*U_b);
I_bdq = I_b*sqrt(2); 
U_bdq = U_b*(sqrt(2/3));

%Current and voltage in pu
v_sd = v_sdq(1)/U_bdq; % input in SI that is coverted to pu
v_sq = v_sdq(2)/U_bdq; % input in SI that is coverted to pu
i_sd = i_sdq(1)/I_bdq; % input in SI that is coverted to pu
i_sq = i_sdq(2)/I_bdq; % input in SI that is coverted to pu
%Active power en pu
p_s = i_sd*v_sd + i_sq*v_sq; % pu
q_s = i_sd*v_sq - i_sq*v_sd; % pu 

% from the integrator to the states
phi  = x(1);
xi_p = x(2);
xi_q = x(3);
omega_fil = x(4);

%error of active and reactive power
epsilon_p = (p_m_ref - p_s)*(1.0-fault_flag);
epsilon_q = q_s_ref - q_s;

%omega VSG
omega = K_p*(epsilon_p + xi_p/T_p) + omega_base; 
omega_rads = 2.0*pi*50.0*omega;
%Derivative outputs
dphi =  omega_rads;
dxi_p = epsilon_p;
dxi_q = epsilon_q; 
domega_rads = 1.0/1.0*(2.0*pi*50.0*omega - omega_fil);

%Voltage increase
DV =   K_q*(epsilon_q + xi_q/T_q); 

%Saturation of DV
DV_sat = DV;
if DV_sat > 0.1 
    DV_sat = 0.1;
    dxi_q = 0.0;
end
if DV_sat < -0.1 
    DV_sat = -0.1;
    dxi_q = 0.0;
end   

%Electromotive force of VSG
e = e_0 + DV_sat; 

%Virtual impdance
i_sd = -(X*e + R*v_sd + X*v_sq)/(R^2 + X^2);
i_sq = -(R*e + R*v_sq - X*v_sd)/(R^2 + X^2);

%Current references in A
i_sdq_ref(1) = i_sd*I_bdq;
i_sdq_ref(2) = i_sq*I_bdq;


% from derivatives to the integrator
dx = [dphi;dxi_p;dxi_q;domega_rads];

== matlab function PI_VC_vs_UPI_CC_3ph_4w_v2023b/Control UVSG/Reference Computation/current_computation ==
  data: v_salbe_a input size=2; i_salbe_a_ref output; v_salbe_b input size=2; v_salbe_c input size=2; pa_ref input; qa_ref input; pb_ref input; qb_ref input; pc_ref input; qc_ref input; i_salbe_b_ref output; i_salbe_c_ref output
function [i_salbe_a_ref,i_salbe_b_ref,i_salbe_c_ref] = fcn(v_salbe_a,v_salbe_b,v_salbe_c,pa_ref,qa_ref,pb_ref,qb_ref,pc_ref,qc_ref)

i_sal_a_ref = 2/3*(pa_ref*v_salbe_a(1) + qa_ref*v_salbe_a(2))/(v_salbe_a(1)^2 + v_salbe_a(2)^2);
i_sbe_a_ref = 2/3*(pa_ref*v_salbe_a(2) - qa_ref*v_salbe_a(1))/(v_salbe_a(1)^2 + v_salbe_a(2)^2);
if sqrt(i_sal_a_ref^2 + i_sbe_a_ref^2)>40
    i_sal_a_ref = 0;
    i_sbe_a_ref = 0;
end
i_salbe_a_ref = [i_sal_a_ref;i_sbe_a_ref]*3;


i_sal_b_ref = 2/3*(pb_ref*v_salbe_b(1) + qb_ref*v_salbe_b(2))/(v_salbe_b(1)^2 + v_salbe_b(2)^2);
i_sbe_b_ref = 2/3*(pb_ref*v_salbe_b(2) - qb_ref*v_salbe_b(1))/(v_salbe_b(1)^2 + v_salbe_b(2)^2);
if sqrt(i_sal_b_ref^2 + i_sbe_b_ref^2)>40
    i_sal_b_ref = 0;
    i_sbe_b_ref = 0;
end
i_salbe_b_ref = [i_sal_b_ref;i_sbe_b_ref]*3;

i_sal_c_ref = 2/3*(pc_ref*v_salbe_c(1) + qc_ref*v_salbe_c(2))/(v_salbe_c(1)^2 + v_salbe_c(2)^2);
i_sbe_c_ref = 2/3*(pc_ref*v_salbe_c(2) - qc_ref*v_salbe_c(1))/(v_salbe_c(1)^2 + v_salbe_c(2)^2);
if sqrt(i_sal_c_ref^2 + i_sbe_b_ref^2)>40
    i_sal_c_ref = 0;
    i_sbe_c_ref = 0;
end
i_salbe_c_ref = [i_sal_c_ref;i_sbe_c_ref]*3;

== matlab function PI_VC_vs_UPI_CC_3ph_4w_v2023b/Measurements UVSG/MATLAB Function ==
  data: i_sabc input; pa output; v_sabc input; qa output; pb output; qb output; pc output; qc output
function [pa,qa,pb,qb,pc,qc] = fcn(i_sabc,v_sabc)

ia = i_sabc(1);
ib = i_sabc(2);
ic = i_sabc(3);

va = v_sabc(1);
vb = v_sabc(2);
vc = v_sabc(3);

pa = ia*va;
qa = 1/sqrt(3)*ia*(vb - vc);

pb = ib*vb;
qb = 1/sqrt(3)*ib*(vc -va);

pc = ic*vc;
qc = 1/sqrt(3)*ic*(va -vb);

== matlab function PI_VC_vs_UPI_CC_3ph_4w_v2023b/Measurements UVSG/power computation ==
  data: i_salbe input; p_s output; q_s output; v_salbe input; params input
function [p_s,q_s] = ctrl_3(i_salbe,v_salbe,params)
S_b = params(1);
U_b = params(2);

I_b = S_b/(sqrt(3)*U_b);
I_bdq = I_b*sqrt(2); 

U_bdq = U_b*(sqrt(2/3));

i_sal = i_salbe(1)/I_bdq; % input in SI that is coverted to pu
i_sbe = i_salbe(2)/I_bdq; % input in SI that is coverted to pu
v_sal = v_salbe(1)/U_bdq; % input in SI that is coverted to pu
v_sbe = v_salbe(2)/U_bdq; % input in SI that is coverted to pu

p_s = i_sal*v_sal + i_sbe*v_sbe; % pu
q_s = i_sal*v_sbe - i_sbe*v_sal; % pu

== matlab function PI_VC_vs_UPI_CC_3ph_4w_v2023b/Control UVSG/Reference Computation/MATLAB Function ==
  data: i_s_abc input; i_s_abc_ref output; time input
function i_s_abc_ref = fcn(i_s_abc,time)
i_s_abc_ref = [0;0;0];

if time >1
    i_s_abc_ref = [i_s_abc(1);i_s_abc(2);i_s_abc(3)];
end

== matlab function PI_VC_vs_UPI_CC_3ph_4w_v2023b/Control PI_VC/MATLAB Function3 ==
  data: theta input size=1; dq output; abc input
function dq  = fcn(theta,abc)
%#codegen

T_p = 2.0/3.0*[[ cos(theta), cos(theta-2.0/3.0*pi), cos(theta+2.0/3.0*pi)];
               [-sin(theta),-sin(theta-2.0/3.0*pi),-sin(theta+2.0/3.0*pi)]];
           
dq=T_p*abc;

== matlab function PI_VC_vs_UPI_CC_3ph_4w_v2023b/Control PI_VC/MATLAB Function4 ==
  data: theta input size=1; dq output; abc input
function dq  = fcn(theta,abc)
%#codegen

T_p = 2.0/3.0*[[ cos(theta), cos(theta-2.0/3.0*pi), cos(theta+2.0/3.0*pi)];
               [-sin(theta),-sin(theta-2.0/3.0*pi),-sin(theta+2.0/3.0*pi)]];
           
dq=T_p*abc;

== matlab function PI_VC_vs_UPI_CC_3ph_4w_v2023b/Control PI_VC/MATLAB Function5 ==
  data: theta input size=1; abc output size=3; dq input
function abc  = fcn(theta,dq)
%#codegen

T_p_inv = [[            cos(theta),            -sin(theta)];
           [ cos(theta-2.0/3.0*pi), -sin(theta-2.0/3.0*pi)];
           [ cos(theta+2.0/3.0*pi), -sin(theta+2.0/3.0*pi)]];
           
abc=T_p_inv*dq;

== matlab function PI_VC_vs_UPI_CC_3ph_4w_v2023b/Control PI_VC/MATLAB Function1 ==
  data: theta input size=1; dq output; abc input
function dq  = fcn(theta,abc)
%#codegen

T_p = 2.0/3.0*[[ cos(theta), cos(theta-2.0/3.0*pi), cos(theta+2.0/3.0*pi)];
               [-sin(theta),-sin(theta-2.0/3.0*pi),-sin(theta+2.0/3.0*pi)]];
           
dq=T_p*abc;

== matlab function PI_VC_vs_UPI_CC_3ph_4w_v2023b/Control PI_VC/MATLAB Function2 ==
  data: theta input size=1; dq output; abc input
function dq  = fcn(theta,abc)
%#codegen

T_p = 2.0/3.0*[[ cos(theta), cos(theta-2.0/3.0*pi), cos(theta+2.0/3.0*pi)];
               [-sin(theta),-sin(theta-2.0/3.0*pi),-sin(theta+2.0/3.0*pi)]];
           
dq=T_p*abc;
